simulink model "SPWM"  (R2019b)
settings: Solver=ode45  StartTime=0.0  StopTime=2  MaxStep=1e-6  RelTol=1e-3
libraries: powerlib x14, simulink x1
Description:
  | SPWM，正弦脉宽调制
settings Model: Creator=DELL  LastModifiedBy=Inspiron
settings DataIOCC: ReturnWorkspaceOutputs=off
settings DebuggingCC: ArithmeticOperatorsInVariantConditions=warning
settings SFSimCC: SimUseLocalCustomCode=off  CustomCodeUndefinedFunction=UseInterfaceOnly
settings RTWCC: RTWUseLocalCustomCode=off
settings CodeAppCC: StateflowObjectComments=on
settings SimscapeCC: SimscapeNormalizeSystem=off

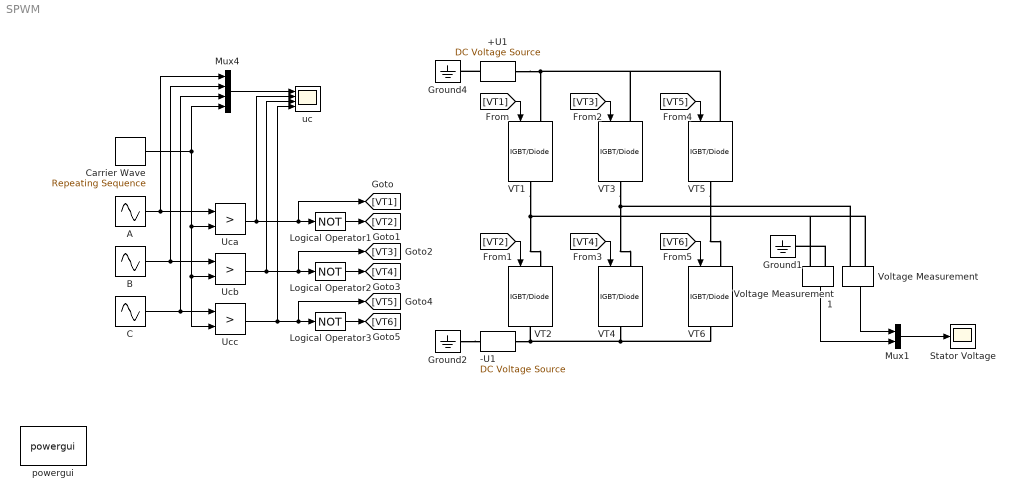
== system SPWM ==
  +U1 : powerlib/Electrical Sources/DC Voltage Source  Amplitude=150  Measurements=None
      settings: SourceProductName=Simscape Electrical
  -U1 : powerlib/Electrical Sources/DC Voltage Source  Amplitude=150  Measurements=None
      settings: SourceProductName=Simscape Electrical
  A : Sin  Frequency=2*pi  SampleTime=0
  B : Sin  Frequency=2*pi  Phase=- 2*pi/3  SampleTime=0
  C : Sin  Frequency=2*pi  Phase=2*pi/3  SampleTime=0
  Carrier Wave : simulink/Sources/Repeating Sequence  rep_seq_t=[0 0.05 0.1]  rep_seq_y=[-1 1 -1]
  Ground1 : powerlib/Elements/Ground  LConnTagsString=a
      settings: SourceProductName=Simscape Electrical
  Ground2 : powerlib/Elements/Ground  LConnTagsString=a
      settings: SourceProductName=Simscape Electrical
  Ground4 : powerlib/Elements/Ground  LConnTagsString=a
      settings: SourceProductName=Simscape Electrical
  Logical Operator1 : Logic  Operator=NOT  AllPortsSameDT=off  OutDataTypeStr=boolean
  Logical Operator2 : Logic  Operator=NOT  AllPortsSameDT=off  OutDataTypeStr=boolean
  Logical Operator3 : Logic  Operator=NOT  AllPortsSameDT=off  OutDataTypeStr=boolean
  Mux1 : Mux  Inputs=2
  Mux4 : Mux
  Stator Voltage : Scope
  Uca : RelationalOperator  Operator=>  OutDataTypeStr=boolean  RndMeth=Simplest
  Ucb : RelationalOperator  Operator=>  OutDataTypeStr=boolean  RndMeth=Simplest
  Ucc : RelationalOperator  Operator=>  OutDataTypeStr=boolean  RndMeth=Simplest
  VT{1..6} (6 alike) : powerlib/Power Electronics/IGBT//Diode  Ron=1e-3  Rs=1e5  Cs=inf  Measurements=off
      settings: SourceProductName=Simscape Electrical
  Voltage Measurement : powerlib/Measurements/Voltage Measurement  PhasorSimulation=off  OutputType=Complex  PSBequivalent=0
      settings: SourceProductName=Simscape Electrical
  Voltage Measurement1 : powerlib/Measurements/Voltage Measurement  PhasorSimulation=off  OutputType=Complex  PSBequivalent=0
      settings: SourceProductName=Simscape Electrical
  powergui : powerlib/powergui  Priority=1  SimulationMode=Continuous  SampleTime=50e-6  frequency=60  Iterations=50  frequencyindice=0  Pbase=100e6  ErrMax=1e-4  UnitsV=kV  UnitsW=MW  buscounter=0  FunctionMessages=off  echomessages=off  EnableUseOfTLC=off  CurrentSourceSwitches=on  DisableSnubberDevices=off  DisableRonSwitches=off  DisableVfSwitches=off  DisplayEquations=off  AutomaticDiscreteSolvers=off  SolverType=Tustin/Backward Euler (TBE)  Interpol=off  ExternalGateDelay=off  methode=off  Ts=10  x0status=blocks  SPID=off  SwTol=0  HookPort=off  NonlinearTolerance=1e-4  nMaxIteration=100  ContinueOnMaxIteration=off  RestoreLinks=warning  ResistiveCurrentMeasurement=off  Frange=[0:2:500]  Ylog=off  Xlog=on  ShowGrid=off  save=off  variable=ZData  structure=0  ZoomFFT=off  StartTime=0.0  cycles=1  DisplayStyle=1  fundamental=60  FreqAxis=off  MaxFrequency=1000  frequencyindicesteady=1  RmsSteady=1  display=off
      settings: SourceProductName=Simscape Electrical
  uc : Scope  NumInputPorts=4
  wires:
  Carrier Wave/1 -> Ucc/2, Ucb/2, Uca/2, Mux4/4
  A/1 -> Mux4/1, Uca/1
  B/1 -> Mux4/2, Ucb/1
  C/1 -> Mux4/3, Ucc/1
  Mux4/1 -> uc/1
  [VT2] -> VT2/1
  Logical Operator1/1 -> [VT2]
  Uca/1 -> [VT1], Logical Operator1/1, uc/2
  [VT1] -> VT1/1
  [VT3] -> VT3/1
  [VT4] -> VT4/1
  [VT5] -> VT5/1
  [VT6] -> VT6/1
  Ucb/1 -> [VT3], Logical Operator2/1, uc/3
  Logical Operator2/1 -> [VT4]
  Ucc/1 -> [VT5], Logical Operator3/1, uc/4
  Logical Operator3/1 -> [VT6]
  Mux1/1 -> Stator Voltage/1
  Voltage Measurement1/1 -> Mux1/2
  Voltage Measurement/1 -> Mux1/1
  connections:
  VT1/RConn1 -- Voltage Measurement/LConn2 -- Voltage Measurement1/LConn1 -- VT2/LConn1
  VT3/RConn1 -- Voltage Measurement/LConn1 -- VT4/LConn1
  VT5/RConn1 -- VT6/LConn1
  +U1/LConn1 -- Ground4/LConn1
  +U1/RConn1 -- VT5/LConn1 -- VT3/LConn1 -- VT1/LConn1
  VT4/RConn1 -- VT6/RConn1 -- -U1/LConn1 -- VT2/RConn1
  Ground2/LConn1 -- -U1/RConn1
  Voltage Measurement1/LConn2 -- Ground1/LConn1
